simulink model "generic_mass_SoC_mu"  (R2025a)
settings: Solver=ode45  StartTime=0.0  StopTime=12  RelTol=1e-3  EnableMultiTasking=on
values from neighbouring files (symbols this model uses):
  Battery =     [Battery_A123_Pack_204s2p_Final.mat]
  cs_tyre = 2.0e5    (= 200000)    [mu_estimator_parameters.m]
  dOCV_dSoC = gradient(OCV, SoC_bp)    [SoCOcv.m]
  dR0 = gradient(R0, SoC_L)    [SoCOcv.m]
  eps_vx = 0.5    [mu_estimator_parameters.m]
  fz_max = 6000    [mu_estimator_parameters.m]
  fz_min = 300    [mu_estimator_parameters.m]
  h_cg = 0.55    [mu_estimator_parameters.m]
  lf = 1.214    [mu_estimator_parameters.m]
  lr = 1.505    [mu_estimator_parameters.m]
  r0 = 0.344    [mu_estimator_parameters.m]
  re_max = 0.33    [mu_estimator_parameters.m]
  re_min = 0.28    [mu_estimator_parameters.m]
  SoC_bp = Table_SoCvsOCV.LUT.SoC_percent    [SoCOcv.m]
  SoC_L = Battery.SOC_LUT    [SoCOcv.m]
  Table_SoCvsOCV = load("SoC_to_Voltage_LUT_10000-GON.mat")    [SoCOcv.m]
  tw_f = 1.571    [mu_estimator_parameters.m]
  tw_r = 1.581    [mu_estimator_parameters.m]
undefined symbols (not defined in the file or in its folder): DiscIntNeverNeededParam, Init_SoC
libraries: CarMaker4SL x41, simulink x1
(part 1 of 4)
settings Model: ModifiedByFormat=IPG  ExtModeAutoUpdateStatusClock=off  VariantFading=off  Creator=IPG  LastModifiedBy=IPG
settings SolverCC: AlgebraicLoopSolver=TrustRegion
settings DataIOCC: LimitDataPoints=on  SaveFormat=Array  SignalLoggingSaveFormat=ModelDataLogs  ReturnWorkspaceOutputs=off  SignalLoggingName=sigsOut
settings OptimizationCC: BooleanDataType=off  ReuseModelBlockBuffer=off  ExpressionDepthLimit=2147483647.0  InitFltsAndDblsToZero=on  LifeSpan=inf
settings DebuggingCC: SaveWithParameterizedLinksMsg=none  UnderspecifiedInitializationDetection=Classic  MergeDetectMultiDrivingBlocksExec=none  SignalResolutionControl=TryResolveAllWithWarning  MultiTaskDSMMsg=warning  MultiTaskCondExecSysMsg=none  FcnCallInpInsideContextMsg=warning  UnconnectedInputMsg=warning  UnconnectedOutputMsg=warning  UnconnectedLineMsg=warning  StateNameClashWarn=warning  SFUnexpectedBacktrackingDiag=warning  SFNoUnconditionalDefaultTransitionDiag=warning  ArithmeticOperatorsInVariantConditions=warning
settings HardwareCC: ProdBitPerPointer=32.0  ProdBitPerSizeT=32.0  ProdBitPerPtrDiffT=32.0  ProdLargestAtomicFloat=None  ProdIntDivRoundTo=Undefined  ProdEndianess=Unspecified  ProdWordSize=32.0  ProdHWDeviceType=32-bit Generic  TargetUnknown=on
settings ModelReferenceCC: EnableRefExpFcnMdlSchedulingChecks=on  PropagateSignalLabelsOutOfModel=off
settings SFSimCC: SimUseLocalCustomCode=off  CustomCodeUndefinedFunction=UseInterfaceOnly
settings RTWCC: RTWUseLocalCustomCode=off  GPUComputeCapability=3.5  DLArmComputeVersion=19.05
settings CodeAppCC: MaxIdLength=63.0  StateflowObjectComments=on
settings GRTTargetCC: TargetFcnLib=ansi_tfl_tmw.mat  TargetLangStandard=C89/C90 (ANSI)  CombineOutputUpdateFcns=off  GRTInterface=on
settings ConfigComp: CovMetricSettings=dw  CovSaveCumulativeToWorkspaceVar=on  CovSaveSingleToWorkspaceVar=on  CovExternalEMLEnable=off

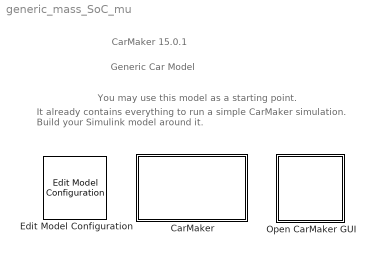
== system generic_mass_SoC_mu ==
  note: Generic Car Model
  note: You may use this model as a starting point.
  note: It already contains everything to run a simple CarMaker simulation.
      | Build your Simulink model around it.
  note: CarMaker 15.0.1
  CarMaker : Subsystem  TreatAsAtomicUnit=on
      mask Display: image(imread('CarMakerSys.png'));
  Edit Model Configuration : CarMaker4SL/Edit Model Configuration  SFunctionModules=''
  Open CarMaker GUI : Subsystem  LoadFcn=if ~length(which('cmself')), cmenv; end
      settings: OpenFcn=cmblockmagic('gui_fix_display'); CM_Simulink
      mask Display: image(imread('CarMakerGUI.png'));

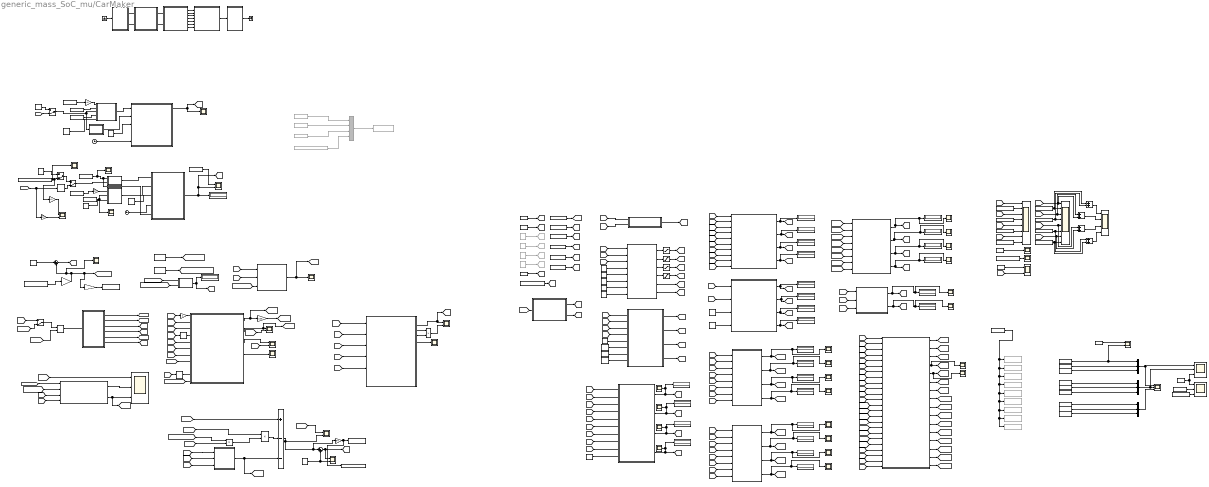
== system generic_mass_SoC_mu/CarMaker ==
  note: Data for Heavy Braking Tests
  note: Heavy Braking Test - Fx Comparison
  note: front_wheel_speed_from_motor
  note: SOC Estimator
  note: Mass and Slop Estimator
  note: Slope Estimator
  note: Mass estimation
  note: Current Input
  note: EXTENDED KALMAN FILTER SOC
  note: Internal resistance estimation
  note: Vt
  note: I.R
  note: Voltage of RC network
  note: ECM MODEL
  note: Terminal
      |  voltage
  note: OCV
  note: INIT
  note: SoC comparison
  note: Cell Capacity Calculation
  note: ECM LOOKUP TABLES
  note: cornering_detector
  note: Mu estimator - Motor Front - 2 Wheels Rear
  note: Outputs
  note: effective_radius_estimator
  note: vertical_load_estimator
  note: Inputs
  note: longitudinal_force_estimator
  note: slip_estimator
  note: mu_combined_estimator
  note: longitudinal_accel_correction
  note: lateral_force_estimator
  note: mu_long_estimator
  note: mu_lat_estimator
  Add : Sum  Inputs=+--
  Add{1..4} (4 alike) : Sum
  Battery total capacity (mAh)2 : Constant  Value=6000
  CM_FIRST : Subsystem
  CM_LAST : Subsystem
  COLOUMB COUNTING : Subsystem
  Clock1 : Clock
  Clock2 : Clock
  Constant : Constant  Value=0.343
  Constant1 : Constant  Value=1770.02
  Constant2 : Constant
  Constant3 : Constant  Value=0.75
  Constant32 : Constant  Value=lf
  Constant33 : Constant  Value=lr
  Constant34 : Constant  Value=h_cg
  Constant35 : Constant  Value=r0
  Constant36 : Constant  Value=cs_tyre
  Constant37 : Constant  Value=re_min
  Constant38 : Constant  Value=re_max
  Constant39 : Constant  Value=eps_vx
  Constant4 : Constant  Value=0
  Constant46 : Constant  Commented=on  Value=1770
  Constant47 : Constant  Commented=on
  Constant48 : Constant  Commented=on  Value=0
  Constant49 : Constant  Value=tw_r
  Constant5 : Constant  Value=1900
  Constant50 : Constant  Value=tw_f
  Constant51 : Constant  Commented=on  Value=0.15
  Constant6 : Constant  Value=0.343
  Constant7 : Constant  Value=lf
  Constant8 : Constant  Value=lr
  Delay : Delay  DelayLength=1  InputProcessing=Columns as channels (frame based)
  Delay1 : Delay  DelayLength=1  InitialConditionSource=Input port  InitialCondition=Init_SoC  InputProcessing=Columns as channels (frame based)
      settings: InputPortMap=u0,p4
  Delay2 : Delay  DelayLength=1  InputProcessing=Columns as channels (frame based)
  Delay3 : Delay  DelayLength=1  InputProcessing=Columns as channels (frame based)
  Display{,1..13,24..37} (28 alike) : Display
  DrivMan : Subsystem
  EKF : MATLAB Function  TreatAsAtomicUnit=on
  Factor internal Resistance : Constant  Value=1.5
  From Workspace : FromWorkspace  VariableName=dryunload
  From Workspace1 : FromWorkspace  VariableName=dryload
  From Workspace2 : FromWorkspace  VariableName=wetunload
  From Workspace3 : FromWorkspace  VariableName=wetload
  From Workspace4 : FromWorkspace  VariableName=dryload1
  From Workspace5 : FromWorkspace  VariableName=wetload1
  From Workspace6 : FromWorkspace  VariableName=iceunload
  From Workspace7 : FromWorkspace  VariableName=iceload
  From Workspace8 : FromWorkspace  VariableName=iceload1
  Gain : Gain  Gain=180/pi
  Gain1 : Gain  Gain=10.65
  Gain2 : Gain  Gain=10.65
  Gain3 : Gain  Gain=180/pi
  Gain4 : Gain  Gain=3/180.9
  Gain5 : Gain  Gain=100
  Gain6 : Gain
  Gain7 : Gain  Gain=94
  Gain8 : Gain  Gain=180.9/3
  Goto112 : Goto  Commented=on  GotoTag=mhat  TagVisibility=global
  Goto123 : Goto  Commented=on  GotoTag=brake  TagVisibility=global
  Goto127 : Goto  Commented=on  GotoTag=throttle  TagVisibility=global
  Goto97 : Goto  Commented=on  GotoTag=beta  TagVisibility=global
  Ground : Ground
  INTERNAL RESISTANCE ESTIMATION : MATLAB Function  TreatAsAtomicUnit=on
  IPG Vehicle : Subsystem
  MATLAB Function : MATLAB Function  TreatAsAtomicUnit=on
  MATLAB Function1 : MATLAB Function  TreatAsAtomicUnit=on
  MATLAB Function17 : MATLAB Function  TreatAsAtomicUnit=on
  MATLAB Function2 : MATLAB Function  TreatAsAtomicUnit=on
  MATLAB Function23 : MATLAB Function  TreatAsAtomicUnit=on
  MATLAB Function24 : MATLAB Function  TreatAsAtomicUnit=on
  MATLAB Function26 : MATLAB Function  TreatAsAtomicUnit=on
  MATLAB Function27 : MATLAB Function  TreatAsAtomicUnit=on
  MATLAB Function28 : MATLAB Function  TreatAsAtomicUnit=on
  MATLAB Function29 : MATLAB Function  TreatAsAtomicUnit=on
  MATLAB Function3 : MATLAB Function  TreatAsAtomicUnit=on
  MATLAB Function30 : MATLAB Function  TreatAsAtomicUnit=on
  MATLAB Function4 : MATLAB Function  TreatAsAtomicUnit=on
  MATLAB Function5 : MATLAB Function  TreatAsAtomicUnit=on
  MATLAB Function6 : MATLAB Function  TreatAsAtomicUnit=on
  MATLAB Function7 : MATLAB Function  TreatAsAtomicUnit=on
  MATLAB Function8 : MATLAB Function  TreatAsAtomicUnit=on
  MATLAB Function9 : MATLAB Function  TreatAsAtomicUnit=on
  Manual Switch{,1..3} (4 alike) : ManualSwitch  CurrentSetting=0
  Mass Estimator : MATLAB Function  TreatAsAtomicUnit=on
  Measurement Error : RandomNumber  Variance=0.00001  Seed=18618  SampleTime=0.01
  Mux : Mux  Inputs=3
  Mux1 : Mux  Inputs=3
  Mux2 : Mux  Inputs=3
  Mux3 : Mux  Commented=on
  Parameter updating : Subsystem
  Process Error : RandomNumber  Variance=0.1  Seed=234513235  SampleTime=0.01
  Product : Product
  Product1 : Product
  RC network subsystem : Subsystem
  Read CM Dict{,3,10,12,25,32} (6 alike) : CarMaker4SL/Read CM Dict  xname=Car.ax  xsync=off  xstime=Continuous
  Read CM Dict1 : CarMaker4SL/Read CM Dict  xname=Car.vx  xsync=off  xstime=Continuous
  Read CM Dict11 : CarMaker4SL/Read CM Dict  xname=Vhcl.FR.rotv  xsync=off  xstime=Continuous
  Read CM Dict13 : CarMaker4SL/Read CM Dict  xname=Vhcl.FL.rotv  xsync=off  xstime=Continuous
  Read CM Dict14 : CarMaker4SL/Read CM Dict  xname=Vhcl.FR.rotv  xsync=off  xstime=Continuous
  Read CM Dict15 : CarMaker4SL/Read CM Dict  xname=Vhcl.RL.rotv  xsync=off  xstime=Continuous
  Read CM Dict16 : CarMaker4SL/Read CM Dict  xname=Vhcl.RR.rotv  xsync=off  xstime=Continuous
  Read CM Dict17 : CarMaker4SL/Read CM Dict  xname=Vhcl.FL.Fz  xsync=off  xstime=Continuous
  Read CM Dict18 : CarMaker4SL/Read CM Dict  xname=PT.Motor.rotv  xsync=off  xstime=Continuous
  Read CM Dict19 : CarMaker4SL/Read CM Dict  xname=Vhcl.FR.Fz  xsync=off  xstime=Continuous
  Read CM Dict2 : CarMaker4SL/Read CM Dict  xname=PT.Motor.Trq  xsync=off  xstime=Continuous
  Read CM Dict20 : CarMaker4SL/Read CM Dict  xname=Vhcl.RL.rotv  xsync=off  xstime=Continuous
  Read CM Dict21 : CarMaker4SL/Read CM Dict  xname=Vhcl.RR.rotv  xsync=off  xstime=Continuous
  Read CM Dict22 : CarMaker4SL/Read CM Dict  xname=Vhcl.RL.Fz  xsync=off  xstime=Continuous
  Read CM Dict23 : CarMaker4SL/Read CM Dict  xname=Vhcl.RR.Fz  xsync=off  xstime=Continuous
  Read CM Dict24 : CarMaker4SL/Read CM Dict  xname=Car.ay  xsync=off  xstime=Continuous
  Read CM Dict26 : CarMaker4SL/Read CM Dict  xname=Car.Road.Route.LongSlope  xsync=off  xstime=Continuous
  Read CM Dict27 : CarMaker4SL/Read CM Dict  xname=Car.Road.Route.LongSlope  xsync=off  xstime=Continuous
  Read CM Dict28 : CarMaker4SL/Read CM Dict  xname=Car.ay  xsync=off  xstime=Continuous
  Read CM Dict29 : CarMaker4SL/Read CM Dict  xname=Vhcl.Steer.Ang  xsync=off  xstime=Continuous
  Read CM Dict30 : CarMaker4SL/Read CM Dict  xname=Car.YawRate  xsync=off  xstime=Continuous
  Read CM Dict31 : CarMaker4SL/Read CM Dict  xname=Car.SideSlipAngle  xsync=off  xstime=Continuous
  Read CM Dict33 : CarMaker4SL/Read CM Dict  xname=Car.vx  xsync=off  xstime=Continuous
  Read CM Dict34 : CarMaker4SL/Read CM Dict  Commented=on  xname=PT.Motor.Trq  xsync=off  xstime=Continuous
  Read CM Dict35 : CarMaker4SL/Read CM Dict  Commented=on  xname=Car.vx  xsync=off  xstime=Continuous
  Read CM Dict36 : CarMaker4SL/Read CM Dict  Commented=on  xname=Car.ax  xsync=off  xstime=Continuous
  Read CM Dict37 : CarMaker4SL/Read CM Dict  Commented=on  xname=Car.Road.Route.LongSlope  xsync=off  xstime=Continuous
  Read CM Dict4 : CarMaker4SL/Read CM Dict  xname=Car.Road.Route.LongSlope  xsync=off  xstime=Continuous
  Read CM Dict5 : CarMaker4SL/Read CM Dict  xname=PT.Motor.Trq  xsync=off  xstime=Continuous
  Read CM Dict6 : CarMaker4SL/Read CM Dict  xname=Car.vx  xsync=off  xstime=Continuous
  Read CM Dict7 : CarMaker4SL/Read CM Dict  xname=Vhcl.FR.Fx  xsync=off  xstime=Continuous
  Read CM Dict8 : CarMaker4SL/Read CM Dict  xname=PT.Motor.Trq  xsync=off  xstime=Continuous
  Read CM Dict9 : CarMaker4SL/Read CM Dict  xname=PT.BattHV.Current  xsync=off  xstime=Continuous
  Saturation{4..7} (4 alike) : Saturate  UpperLimit=fz_max  LowerLimit=fz_min
  Scope{,1..2,4,6,9,13,15..25,29..38,42,44} (30 alike) : Scope
      Scope settings: ActiveDisplayYMinimum=-1  ActiveDisplayYMaximum=1
      Scope1 settings: ActiveDisplayYMinimum=-1  ActiveDisplayYMaximum=1
      Scope13 settings: ActiveDisplayYMinimum=-0.0040490561765422206  ActiveDisplayYMaximum=0.0023870747364762024  DataLoggingVariableName=ScopeData13
      Scope15 settings: ActiveDisplayYMinimum=5.267786429043011  ActiveDisplayYMaximum=6.0813570634396656  DataLoggingVariableName=ScopeData15
      Scope16 settings: ActiveDisplayYMinimum=-0.78309060543519626  ActiveDisplayYMaximum=0.78396172750172144  DataLoggingVariableName=ScopeData18
      Scope17 settings: ActiveDisplayYMinimum=-1  ActiveDisplayYMaximum=1  DataLoggingVariableName=ScopeData19
      Scope18 settings: ActiveDisplayYMinimum=-1  ActiveDisplayYMaximum=1  DataLoggingVariableName=ScopeData20
      Scope19 settings: ActiveDisplayYMinimum=-1  ActiveDisplayYMaximum=1  DataLoggingVariableName=ScopeData21
      Scope2 settings: ActiveDisplayYMinimum=-1  ActiveDisplayYMaximum=1  DataLoggingVariableName=ScopeData2
      Scope20 settings: ActiveDisplayYMinimum=-0.78309060543519626  ActiveDisplayYMaximum=0.78396172750172144  DataLoggingVariableName=ScopeData22
      Scope21 settings: ActiveDisplayYMinimum=-1  ActiveDisplayYMaximum=1  DataLoggingVariableName=ScopeData23
      Scope22 settings: ActiveDisplayYMinimum=-1  ActiveDisplayYMaximum=1  DataLoggingVariableName=ScopeData24
      Scope23 settings: ActiveDisplayYMinimum=-1  ActiveDisplayYMaximum=1  DataLoggingVariableName=ScopeData25
      Scope24 settings: ActiveDisplayYMinimum=-7189.1945849733847  ActiveDisplayYMaximum=6347.4205470208444  DataLoggingVariableName=ScopeData26
      Scope25 settings: ActiveDisplayYMinimum=-3261.1629631477726  ActiveDisplayYMaximum=457.08980839058904  DataLoggingVariableName=ScopeData27
      Scope29 settings: ActiveDisplayYMinimum=-0.092654151933100309  ActiveDisplayYMaximum=0.77993922328861376  DataLoggingVariableName=ScopeData31
      Scope30 settings: ActiveDisplayYMinimum=-1  ActiveDisplayYMaximum=1  DataLoggingVariableName=ScopeData32
      Scope31 settings: ActiveDisplayYMinimum=-1  ActiveDisplayYMaximum=1  DataLoggingVariableName=ScopeData33
      Scope32 settings: ActiveDisplayYMinimum=-1  ActiveDisplayYMaximum=1  DataLoggingVariableName=ScopeData34
      Scope33 settings: DataLoggingVariableName=ScopeData35
      Scope34 settings: DataLoggingVariableName=ScopeData36
      Scope35 settings: DataLoggingVariableName=ScopeData37
      Scope36 settings: DataLoggingVariableName=ScopeData38
      Scope37 settings: ActiveDisplayYMinimum=-1  ActiveDisplayYMaximum=1  DataLoggingVariableName=ScopeData39
      Scope38 settings: ActiveDisplayYMinimum=-0.0655570660830278  ActiveDisplayYMaximum=0.59001359474725035  DataLoggingVariableName=ScopeData40
      Scope4 settings: ActiveDisplayYMinimum=0.17650245012519925  ActiveDisplayYMaximum=0.22445297416691398  DataLoggingVariableName=ScopeData6
      Scope42 settings: ActiveDisplayYMinimum=-1  ActiveDisplayYMaximum=1  DataLoggingVariableName=ScopeData44
      Scope44 settings: ActiveDisplayYMinimum=-1  ActiveDisplayYMaximum=1  DataLoggingVariableName=ScopeData46
      Scope6 settings: ActiveDisplayYMinimum=-7.6253012416574766  ActiveDisplayYMaximum=8.8462173056425879  DataLoggingVariableName=ScopeData4
      Scope9 settings: ActiveDisplayYMinimum=-0.0013929215683664009  ActiveDisplayYMaximum=0.0015298641956065784  DataLoggingVariableName=ScopeData8
  Scope{3,5,7..8,10..12,39,43} (9 alike) : Scope  NumInputPorts=2
      Scope10 settings: ActiveDisplayYMinimum=65.290304256240674  ActiveDisplayYMaximum=81.634785578223827  DataLoggingVariableName=ScopeData12
      Scope11 settings: ActiveDisplayYMinimum=0.0023982019976572207  ActiveDisplayYMaximum=0.002548408512625157  DataLoggingVariableName=ScopeData11
      Scope12 settings: ActiveDisplayYMinimum=-0.56498027572656229  ActiveDisplayYMaximum=4.9570490949911772  DataLoggingVariableName=ScopeData10
      Scope3 settings: ActiveDisplayYMinimum=1671.5980824561561  ActiveDisplayYMaximum=1724.2201262046208  DataLoggingVariableName=ScopeData5
      Scope39 settings: ActiveDisplayYMinimum=-1  ActiveDisplayYMaximum=1  DataLoggingVariableName=ScopeData41
      Scope43 settings: ActiveDisplayYMinimum=-21.798623721322567  ActiveDisplayYMaximum=18.483609956058363  DataLoggingVariableName=ScopeData45
      Scope5 settings: ActiveDisplayYMinimum=1.9265881549094703  ActiveDisplayYMaximum=4.0763345822165622  DataLoggingVariableName=ScopeData3
      Scope7 settings: ActiveDisplayYMinimum=3.7961685683353883  ActiveDisplayYMaximum=4.0277331935579088  DataLoggingVariableName=ScopeData7
      Scope8 settings: ActiveDisplayYMinimum=-0.11005098491461757  ActiveDisplayYMaximum=0.33783186441057322  DataLoggingVariableName=ScopeData9
  Scope{14,26..28} (4 alike) : Scope  NumInputPorts=3
      Scope14 settings: ActiveDisplayYMinimum=77.508392623156581  ActiveDisplayYMaximum=80.277220204122059  DataLoggingVariableName=ScopeData14
      Scope26 settings: ActiveDisplayYMinimum=-6904.8747954168166  ActiveDisplayYMaximum=5352.9283821189529  DataLoggingVariableName=ScopeData28
      Scope27 settings: ActiveDisplayYMinimum=-14.214999613778026  ActiveDisplayYMaximum=6.4649955098955347  DataLoggingVariableName=ScopeData29
      Scope28 settings: ActiveDisplayYMinimum=-10103.459891915962  ActiveDisplayYMaximum=5366.5694146923006  DataLoggingVariableName=ScopeData30
  Scope40 : Scope  NumInputPorts=8
      settings: ActiveDisplayYMinimum=-7.925692503758305  ActiveDisplayYMaximum=71.331065439918262  DataLoggingVariableName=ScopeData42
  Scope41 : Scope  NumInputPorts=8
      settings: ActiveDisplayYMinimum=1521.5777290365256  ActiveDisplayYMaximum=7221.6093076040352  DataLoggingVariableName=ScopeData43
  Scope45 : Scope  NumInputPorts=4
      settings: ActiveDisplayYMinimum=4074.5734716038833  ActiveDisplayYMaximum=14328.60737357984  DataLoggingVariableName=ScopeData47
  Slope estimator : MATLAB Function  TreatAsAtomicUnit=on
  Sum : Sum  Inputs=|++
  Sum2 : Sum  Inputs=|++
  Terminator : Terminator
  To Workspace : ToWorkspace  VariableName=I_cm_real  SaveFormat=Timeseries  SampleTime=-1
  To Workspace1 : ToWorkspace  VariableName=V_cm_real  SaveFormat=Timeseries  SampleTime=-1
  To Workspace10 : ToWorkspace  Commented=on  VariableName=iceload1  SaveFormat=Timeseries  SampleTime=-1
  To Workspace11 : ToWorkspace  Commented=on  VariableName=MK_DataCM  SaveFormat=Timeseries  SampleTime=-1
  To Workspace2 : ToWorkspace  Commented=on  VariableName=dryload  SaveFormat=Timeseries  SampleTime=-1
  To Workspace3 : ToWorkspace  Commented=on  VariableName=dryunload  SaveFormat=Timeseries  SampleTime=-1
  To Workspace4 : ToWorkspace  Commented=on  VariableName=wetunload  SaveFormat=Timeseries  SampleTime=-1
  To Workspace5 : ToWorkspace  Commented=on  VariableName=wetload  SaveFormat=Timeseries  SampleTime=-1
  To Workspace6 : ToWorkspace  Commented=on  VariableName=dryload1  SaveFormat=Timeseries  SampleTime=-1
  To Workspace7 : ToWorkspace  Commented=on  VariableName=wetload1  SaveFormat=Timeseries  SampleTime=-1
  To Workspace8 : ToWorkspace  Commented=on  VariableName=iceload  SaveFormat=Timeseries  SampleTime=-1
  To Workspace9 : ToWorkspace  Commented=on  VariableName=iceunload  SaveFormat=Timeseries  SampleTime=-1
  VehicleControl : Subsystem
  Write CM Dict1 : CarMaker4SL/Write CM Dict  xname=PT.BattHV.Volt_oc  xsync=off
  multiply : Product  Inputs=**
  tag scope: HL=global, R0=global, Uoc=global, ax=global, ax_eff=global, ay=global, corner=global, dUoc_dSoc=global, fx_fl=global, fx_fr=global, fx_front=global, fx_rear=global, fx_rl=global, fx_rr=global, fy_fl=global, fy_fr=global, fy_front=global, fy_rear=global, fy_rl=global, fy_rr=global, fz_fl=global, fz_fr=global, fz_front=global, fz_rear=global, fz_rl=global, fz_rr=global, mu=global, mu_fl=global, mu_fr=global, mu_front=global, mu_lat=global, mu_lat_fl=global, mu_lat_fr=global, mu_lat_front=global, mu_lat_rear=global, mu_lat_rl=global, mu_lat_rr=global, mu_long=global, mu_long_fl=global, mu_long_fr=global, mu_long_front=global, mu_long_rear=global, mu_long_rl=global, mu_long_rr=global, mu_rear=global, mu_rl=global, mu_rr=global, om_fl=global, om_fr=global, om_front=global, om_rl=global, om_rr=global, re_fl=global, re_fr=global, re_rl=global, re_rr=global, slip=global, slipAng=global, slip_fl=global, slip_fr=global, slip_front=global, slip_rear=global, slip_rl=global, slip_rr=global, slope=global, steer=global, vx=global, yaw_r=global
  wires:
  DrivMan/2(DrivMan.Out) -> VehicleControl/2(DrivMan.In)
  DrivMan/1(Sync_Out) -> VehicleControl/1(Sync_In)
  CM_FIRST/2(Env.Misc) -> DrivMan/2(Env.Misc)
  CM_FIRST/1(Sync_Out) -> DrivMan/1(Sync_In)
  CM_LAST/1(Sync_Out) -> Terminator/1
  Ground/1 -> CM_FIRST/1(Sync_In)
  IPG Vehicle/1(Sync_Out) -> CM_LAST/1(Sync_In)
  VehicleControl/1(Sync_Out) -> IPG Vehicle/1(Sync_In)
  VehicleControl/3(VhclCtrl.Steering) -> IPG Vehicle/3(VhclCtrl.Steering)
  VehicleControl/4(Vhcl.Wheel.In) -> IPG Vehicle/4(Vhcl.Wheel.In)
  VehicleControl/5(Vhcl.Misc) -> IPG Vehicle/5(Vhcl.Misc)
  VehicleControl/6(VhclCtrl.Brake) -> IPG Vehicle/6(VhclCtrl.Brake)
  VehicleControl/7(VhclCtrl.PT) -> IPG Vehicle/7(VhclCtrl.PT)
  VehicleControl/2(Vhcl.Model.Source) -> IPG Vehicle/2(Vhcl.Model.Source)
  [mhat] -> Manual Switch2/2
  Read CM Dict2/1 -> Gain2/1
  Slope estimator/1(theta2_hat) -> Scope4/1, [beta]
  Constant3/1 -> Slope estimator/3(lambda2)
  Constant5/1 -> Manual Switch2/1
  Manual Switch2/1 -> MATLAB Function5/3(mhat), MATLAB Function6/1(mhat)
  Read CM Dict1/1 -> MATLAB Function5/2(vx)
  MATLAB Function5/1(y2) -> Slope estimator/1(y2)
  Clock1/1 -> Slope estimator/5(t)
  MATLAB Function6/1(phi2) -> Slope estimator/2(phi2)
  Read CM Dict/1 -> MATLAB Function5/4(ax)
  Clock2/1 -> Mass Estimator/4(t)
  Manual Switch/1 -> MATLAB Function2/2(beta)
  Read CM Dict4/1 -> Scope1/1, Gain3/1, Manual Switch1/2
  Mass Estimator/1(m_hat) -> [mhat], Scope3/2, Display/1
  Constant4/1 -> Manual Switch1/1
  MATLAB Function3/1(phi) -> Mass Estimator/2(phi)
  Read CM Dict5/1 -> Gain1/1
  Delay/1 -> Manual Switch/2
  Constant2/1 -> Mass Estimator/3(lambda)
  Manual Switch1/1 -> Manual Switch/1
  Read CM Dict6/1 -> Scope/1, MATLAB Function3/2(vx)
  MATLAB Function2/1(y) -> Mass Estimator/1(y)
  [beta] -> Gain/1, Delay/1
  Read CM Dict3/1 -> Scope2/1, Mass Estimator/5(ax), MATLAB Function2/1(ax)
  Gain1/1 -> MATLAB Function3/1(T_tq)
  Gain2/1 -> MATLAB Function5/1(Tq)
  Constant1/1 -> Scope3/1
  Constant6/1 -> MATLAB Function3/3(re)
  Gain/1 -> Scope5/2
  Gain3/1 -> Scope5/1
  Sum2/1 -> [Current]
  Read CM Dict9/1 -> Gain4/1
  Gain4/1 -> Scope6/1, Sum2/2, Gain8/1, [current_real]
  Process Error/1 -> Sum2/1
  [Vp_real] -> Scope8/2  "Vp_real"
  [Uoc] -> EKF/3(Uoc)
  EKF/3(ul_hat) -> Scope7/1  "vt_hat"
  Delay2/1 -> EKF/10(Qcap_est)
  [Vt] -> EKF/2(UL_meas)
  [R0] -> EKF/5(R0nom)
  EKF/2(u1_hat) -> [u1_hat], Scope8/1  "Vp_hat"
  INTERNAL RESISTANCE ESTIMATION/2(innov_theta) -> Scope13/1
  [MaxBatteryCap] -> EKF/11(Qnom)
  [Uoc] -> INTERNAL RESISTANCE ESTIMATION/3(Uoc)
  [C1] -> EKF/7(C1)
  [R0] -> Product1/1
  [Vt] -> Scope7/2  "vt_real"
  Delay3/1 -> EKF/4(R0_est)
  EKF/4(innov) -> Scope9/1
  Gain6/1 -> EKF/1(I)
  [Current] -> Gain6/1
  [u1_hat] -> INTERNAL RESISTANCE ESTIMATION/5(u1_hat)
  [R0] -> INTERNAL RESISTANCE ESTIMATION/4(R0_init)
  [Vt] -> INTERNAL RESISTANCE ESTIMATION/2(UL_meas)
  Product1/1 -> Scope11/2  "real_R0"
  INTERNAL RESISTANCE ESTIMATION/1(R0_hat) -> [R0_hat], Scope11/1  "R0 hat"
  [dUoc_dSoc] -> EKF/8(dUoc_dSoc)
  [Facto_Internal_Resistance] -> Product1/2
  [R0_hat] -> Delay3/1
  [R1] -> EKF/6(R1)
  Gain5/1 -> [SoC]
  [Q_est] -> Delay2/1
  EKF/1(soc_hat) -> [SoC_hat], Gain5/1
  [Current] -> INTERNAL RESISTANCE ESTIMATION/1(I)
  [C1] -> RC network subsystem/3(" C1")
  Product/1 -> multiply/2
  [R1] -> RC network subsystem/2(R1)
  [current_real] -> multiply/1
  [Facto_Internal_Resistance] -> Product/1
  [Uoc] -> Add/1
  Add/1 -> Gain7/1, Sum/1, Scope10/2
  [R0] -> Product/2
  [current_real] -> RC network subsystem/1(current (A))
  Measurement Error/1 -> Sum/2, Scope12/2
  RC network subsystem/1(V1) -> [Vp_real], Add/3
  multiply/1 -> Add/2
  [SoC] -> Scope10/1
  MATLAB Function4/1(Q_real) -> [Q_real], Display1/1
  [Facto_Internal_Resistance] -> MATLAB Function4/2(factor_internal_resistance)
  Factor internal Resistance/1 -> [Facto_Internal_Resistance]
  [MaxBatteryCap] -> MATLAB Function4/1(Qmax)
  Battery total capacity (mAh)2/1 -> [MaxBatteryCap]
  [Q_real] -> COLOUMB COUNTING/4(Q_real)
  COLOUMB COUNTING/2(Col COUNT) -> Scope14/3, [SoC_Col]  "Coloumb Counting"
  [MaxBatteryCap] -> COLOUMB COUNTING/2(Qmax)
  [current_real] -> COLOUMB COUNTING/1(current real)
  [SoC] -> Scope14/1  "EKF"
  [Current] -> COLOUMB COUNTING/3(current real1)
  COLOUMB COUNTING/1(Real Soc) -> Scope14/2  "Real SoC"
  MATLAB Function/1(C_batt) -> [Q_est], Scope15/1
  [MaxBatteryCap] -> MATLAB Function/3(C_init)
  [R0] -> MATLAB Function/2(R_init)
  [R0_hat] -> MATLAB Function/1(R_batt)
  Gain8/1 -> To Workspace/1
  Sum/1 -> Scope12/1, [Vt]
  Parameter updating/2(Ro) -> [R0]
  Manual Switch3/1 -> Delay1/1
  Parameter updating/1(Voc) -> [Uoc]
  Parameter updating/4(C1) -> [C1]
  [SoC_Col] -> Manual Switch3/2
  Delay1/1 -> Parameter updating/1(SoC)
  [SoC] -> Manual Switch3/1
  Parameter updating/6(dR0) -> [dR0]
  Parameter updating/5(dVoc) -> [dUoc_dSoc]
  [Init_SoC] -> Delay1/2
  Parameter updating/3(R1) -> [R1]
  Gain7/1 -> Write CM Dict1/1, To Workspace1/1
  Constant/1 -> MATLAB Function5/5(re)
  Read CM Dict29/1 -> [steer]
  Read CM Dict31/1 -> [slipAng]
  Read CM Dict30/1 -> [yaw_r]
  Read CM Dict28/1 -> [ay]
  MATLAB Function27/2(high_lateral_flag) -> [HL], Display29/1, Scope38/1
  MATLAB Function27/1(cornering_flag) -> [corner], Display28/1, Scope37/1
  [ay] -> MATLAB Function27/1(steer)
  [slipAng] -> MATLAB Function27/2(ay)
  [steer] -> MATLAB Function27/3(slip_angle)
  Read CM Dict18/1 -> [om_front]
  Read CM Dict20/1 -> [om_rl]
  Read CM Dict21/1 -> [om_rr]
  Read CM Dict33/1 -> [vx]
  Read CM Dict32/1 -> [ax]
  [fz_rl] -> MATLAB Function29/3(fz_rl)
  [re_fr] -> MATLAB Function30/7(re_fr)
  [slip_rl] -> MATLAB Function26/3(slip_rl)
  MATLAB Function26/2(slip_rear_avg) -> [slip_rear]
  Constant46/1 -> Goto112/1
  Constant51/1 -> Goto97/1
  Constant48/1 -> Goto127/1
  Constant39/1 -> MATLAB Function30/10(eps_vx)
  Constant47/1 -> Goto123/1
  Saturation4/1 -> [fz_fl]
  MATLAB Function26/8(mu_long_front_avg) -> [mu_long_front]
  [re_rl] -> MATLAB Function30/8(re_rl)
  Constant38/1 -> MATLAB Function29/8(re_max)
  [ax] -> MATLAB Function17/1(ax)
  MATLAB Function17/1(ax_eff) -> [ax_eff]
  [gas] -> MATLAB Function23/10(throttle_cmd)
  [slip_rr] -> MATLAB Function26/4(slip_rr)
  [re_rr] -> MATLAB Function30/9(re_rr)
  [mu_long_rr] -> MATLAB Function24/4(mu_long_rr)
  MATLAB Function23/4(fx_rr) -> Display25/1, [fx_rr]
  [slip_fl] -> MATLAB Function26/1(slip_fl)
  Saturation6/1 -> [fz_rl]
  MATLAB Function30/1(slip_fl) -> [slip_fl], Display34/1, Scope36/1
  MATLAB Function23/3(fx_rl) -> Display24/1, [fx_rl]
  MATLAB Function23/2(fx_fr) -> Display27/1, [fx_fr]
  MATLAB Function26/7(fy_rear_total) -> [fy_rear]
  [vx] -> MATLAB Function30/5(omega_rr)
  [slip_fr] -> MATLAB Function26/2(slip_fr)
  MATLAB Function24/4(mu_comb_rr) -> [mu_rr], Display33/1, Scope32/1
  Saturation7/1 -> [fz_rr]
  Saturation5/1 -> [fz_fr]
  [mu_long_rl] -> MATLAB Function24/3(mu_long_rl)
  [mu_long_fl] -> MATLAB Function24/1(mu_long_fl)
  Constant35/1 -> MATLAB Function29/5(r0)
  [fz_fl] -> MATLAB Function29/1(fz_fl)
  [fz_rr] -> MATLAB Function29/4(fz_rr)
  Constant37/1 -> MATLAB Function29/7(re_min)
  [fz_fr] -> MATLAB Function29/2(fz_fr)
  Constant36/1 -> MATLAB Function29/6(cs_tyre)
  MATLAB Function30/3(slip_rl) -> [slip_rl], Display35/1, Scope34/1
  [om_fl] -> MATLAB Function30/1(vx)
  [mu_lat_rl] -> MATLAB Function24/7(mu_lat_rl)
  MATLAB Function26/3(slip_vehicle_avg) -> [slip]
  MATLAB Function29/1(re_fl) -> [re_fl]
  MATLAB Function29/4(re_rr) -> [re_rr]
  MATLAB Function26/6(fy_front_total) -> [fy_front]
  MATLAB Function29/3(re_rl) -> [re_rl]
  [om_rr] -> MATLAB Function30/4(omega_rl)
  MATLAB Function29/2(re_fr) -> [re_fr]
  MATLAB Function23/1(fx_fl) -> Display26/1, [fx_fl]
  MATLAB Function24/1(mu_comb_fl) -> [mu_fl], Display30/1, Scope29/1
  [re_fl] -> MATLAB Function30/6(re_fl)
  MATLAB Function24/3(mu_comb_rl) -> [mu_rl], Display32/1, Scope31/1
  [brake] -> MATLAB Function23/9(brake_cmd)
  [om_fr] -> MATLAB Function30/2(omega_fl)
  [om_rl] -> MATLAB Function30/3(omega_fr)
  MATLAB Function24/2(mu_comb_fr) -> [mu_fr], Display31/1, Scope30/1
  MATLAB Function30/2(slip_fr) -> [slip_fr], Display37/1, Scope35/1
  MATLAB Function30/4(slip_rr) -> [slip_rr], Display36/1, Scope33/1
  MATLAB Function26/1(slip_front_avg) -> [slip_front]
  MATLAB Function26/5(fx_rear_total) -> Scope25/1, [fx_rear]
  [mu_long_fr] -> MATLAB Function24/2(mu_long_fr)
  [mu_lat_rr] -> MATLAB Function24/8(mu_lat_rr)
  MATLAB Function26/10(mu_long_vehicle_avg) -> [mu_long]
  MATLAB Function26/9(mu_long_rear_avg) -> [mu_long_rear]
  [mu_lat_fl] -> MATLAB Function24/5(mu_lat_fl)
  [mu_lat_fr] -> MATLAB Function24/6(mu_lat_fr)
  [om_front] -> MATLAB Function1/1(omega_motor_f)
  MATLAB Function1/1(omega_fl) -> [om_fl]
  MATLAB Function1/2(omega_fr) -> [om_fr]
  Constant7/1 -> MATLAB Function7/3(lf)
  MATLAB Function7/1(fy_fl) -> Display4/1, [fy_fl]
  MATLAB Function7/2(fy_fr) -> Display5/1, [fy_fr]
  MATLAB Function7/3(fy_rl) -> Display2/1, [fy_rl]
  [ax_eff] -> MATLAB Function7/2(ay)
  MATLAB Function7/4(fy_rr) -> [fy_rr], Display3/1
  Constant8/1 -> MATLAB Function7/4(lr)
  [mhat] -> MATLAB Function7/1(mhat)
  [fx_fr] -> MATLAB Function8/2(fx_fr)
  [fx_fl] -> MATLAB Function8/1(fx_fl)
  [fx_rr] -> MATLAB Function8/4(fx_rr)
  [fz_fr] -> MATLAB Function8/6(fz_fr)
  MATLAB Function8/2(mu_long_fr) -> Scope17/1, Display7/1, [mu_long_fr]
  MATLAB Function8/3(mu_long_rl) -> Scope18/1, Display8/1, [mu_long_rl]
  MATLAB Function8/1(mu_long_fl) -> Scope16/1, Display6/1, [mu_long_fl]
  [fx_rl] -> MATLAB Function8/3(fx_rl)
  [fz_fl] -> MATLAB Function8/5(fz_fl)
  [fz_rl] -> MATLAB Function8/7(fz_rl)
  MATLAB Function8/4(mu_long_rr) -> Scope19/1, Display9/1, [mu_long_rr]
  [fz_rr] -> MATLAB Function8/8(fz_rr)
  [fz_rr] -> MATLAB Function9/8(fz_rr)
  MATLAB Function9/4(mu_lat_rr) -> [mu_lat_rr], Display13/1, Scope23/1
  [fz_rl] -> MATLAB Function9/7(fz_rl)
  [fz_fl] -> MATLAB Function9/5(fz_fl)
  [fy_rl] -> MATLAB Function9/3(fy_rl)
  MATLAB Function9/1(mu_lat_fl) -> [mu_lat_fl], Display10/1, Scope20/1
  MATLAB Function9/3(mu_lat_rl) -> [mu_lat_rl], Display12/1, Scope22/1
  MATLAB Function9/2(mu_lat_fr) -> [mu_lat_fr], Display11/1, Scope21/1
  [fz_fr] -> MATLAB Function9/6(fz_fr)
  [fy_rr] -> MATLAB Function9/4(fy_rr)
  [fy_fl] -> MATLAB Function9/1(fy_fl)
  [fy_fr] -> MATLAB Function9/2(fy_fr)
  [fx_fl] -> MATLAB Function26/5(fx_fl)
  [fx_fr] -> MATLAB Function26/6(fx_fr)
  [fx_rl] -> MATLAB Function26/7(fx_rl)
  [fx_rr] -> MATLAB Function26/8(fx_rr)
  [fy_fl] -> MATLAB Function26/9(fy_fl)
  [fy_fr] -> MATLAB Function26/10(fy_fr)
  [fy_rl] -> MATLAB Function26/11(fy_rl)
  [fy_rr] -> MATLAB Function26/12(fy_rr)
  [mu_fl] -> MATLAB Function26/21(mu_comb_fl)
  [mu_fr] -> MATLAB Function26/22(mu_comb_fr)
  [mu_rl] -> MATLAB Function26/23(mu_comb_rl)
  [mu_rr] -> MATLAB Function26/24(mu_comb_rr)
  [mu_long_fl] -> MATLAB Function26/13(mu_long_fl)
  [mu_long_fr] -> MATLAB Function26/14(mu_long_fr)
  [mu_long_rl] -> MATLAB Function26/15(mu_long_rl)
  [mu_long_rr] -> MATLAB Function26/16(mu_long_rr)
  [mu_lat_rr] -> MATLAB Function26/20(mu_lat_rr)
  [mu_lat_rl] -> MATLAB Function26/19(mu_lat_rl)
  [mu_lat_fr] -> MATLAB Function26/18(mu_lat_fr)
  [mu_lat_fl] -> MATLAB Function26/17(mu_lat_fl)
  MATLAB Function26/11(mu_lat_front_avg) -> [mu_lat_front]
  MATLAB Function26/12(mu_lat_rear_avg) -> [mu_lat_rear]
  MATLAB Function26/13(mu_lat_vehicle_avg) -> [mu_lat]
  MATLAB Function26/16(mu_comb_vehicle_avg) -> [mu]
  MATLAB Function26/15(mu_comb_rear_avg) -> [mu_rear]
  MATLAB Function26/14(mu_comb_front_avg) -> [mu_front]
  From Workspace/1 -> Scope39/2, Mux/1  "dry_unload"
  From Workspace1/1 -> Mux/2  "dry_load_400kg"
  From Workspace2/1 -> Mux1/1  "wet_unload"
  From Workspace3/1 -> Mux1/2  "wet_load_400kg"
  MATLAB Function26/4(fx_front_total) -> Scope24/1, [fx_front]
  From Workspace4/1 -> Mux/3  "dry_load_600kg"
  From Workspace5/1 -> Mux1/3  "wet_load_600kg"
  From Workspace6/1 -> Mux2/1  "ice_unload"
  From Workspace7/1 -> Mux2/2  "ice_load_400kg"
  From Workspace8/1 -> Mux2/3  "ice_load_600kg"
  Mux/1 -> Scope28/1, Scope26/1
  Mux1/1 -> Scope26/2, Scope28/2
  Mux2/1 -> Scope28/3
  Read CM Dict7/1 -> To Workspace2/1, To Workspace4/1, To Workspace5/1, To Workspace6/1, To Workspace7/1, To Workspace10/1, To Workspace8/1, To Workspace9/1, To Workspace3/1
  Read CM Dict10/1 -> Scope26/3, Scope27/1  "ax"
  Read CM Dict8/1 -> Scope27/2
  Read CM Dict11/1 -> Scope27/3
  Read CM Dict12/1 -> Scope39/1  "ax"
  [fz_rl] -> MATLAB Function23/7(fz_rl)
  [fz_rr] -> MATLAB Function23/8(fz_rr)
  [fz_fr] -> MATLAB Function23/6(fz_fr)
  [fz_fl] -> MATLAB Function23/5(fz_fl)
  [slip_fl] -> MATLAB Function23/1(slip_fl)
  [slip_fr] -> MATLAB Function23/2(slip_fr)
  [slip_rr] -> MATLAB Function23/4(slip_rr)
  [slip_rl] -> MATLAB Function23/3(slip_rl)
  [om_fl] -> Scope40/1  "om_fl"
  Read CM Dict13/1 -> Scope40/2  "fl"
  [om_fr] -> Scope40/3  "om_fr"
  Read CM Dict14/1 -> Scope40/4  "fr"
  [om_rl] -> Scope40/5  "om_rl"
  Read CM Dict15/1 -> Scope40/6  "rl"
  [om_rr] -> Scope40/7  "om_rr"
  Read CM Dict16/1 -> Scope40/8  "rr"
  Read CM Dict23/1 -> Add4/2, Scope41/8  "rr"
  [fz_rr] -> Scope41/7, Add2/2  "fz_rr"
  Read CM Dict22/1 -> Add4/1, Scope41/6  "rl"
  [fz_rl] -> Add2/1, Scope41/5  "fz_rl"
  Read CM Dict19/1 -> Add3/2, Scope41/4  "fr"
  [fz_fr] -> Add1/1, Scope41/3  "fz_fr"
  Read CM Dict17/1 -> Add3/1, Scope41/2  "fl"
  [fz_fl] -> Add1/2, Scope41/1  "fz_fl"
  Read CM Dict24/1 -> Scope42/1
  Read CM Dict25/1 -> Scope43/1
  [ax_eff] -> Scope43/2  "ax_eff"
  Read CM Dict26/1 -> [slope]
  [slope] -> MATLAB Function17/2(slope)
  Read CM Dict27/1 -> Scope44/1
  Add3/1 -> Scope45/1  "front_CM"
  Add1/1 -> Scope45/2  "front_est"
  Add2/1 -> Scope45/3  "rear_est"
  Add4/1 -> Scope45/4  "rear_CM"
  [mhat] -> MATLAB Function28/1(mhat)
  [ax_eff] -> MATLAB Function28/2(ax_eff)
  [ay] -> MATLAB Function28/3(ay)
  Constant32/1 -> MATLAB Function28/4(lf)
  Constant33/1 -> MATLAB Function28/5(lr)
  Constant34/1 -> MATLAB Function28/6(h_cg)
  Constant50/1 -> MATLAB Function28/7(tw_f)
  Constant49/1 -> MATLAB Function28/8(tw_r)
  MATLAB Function28/1(fz_fl) -> Saturation4/1
  MATLAB Function28/2(fz_fr) -> Saturation5/1
  MATLAB Function28/3(fz_rl) -> Saturation6/1
  MATLAB Function28/4(fz_rr) -> Saturation7/1
  MATLAB Function28/5(fz_front_total) -> [fz_front]
  MATLAB Function28/6(fz_rear_total) -> [fz_rear]
  Read CM Dict34/1 -> Mux3/1
  Read CM Dict35/1 -> Mux3/2
  Read CM Dict36/1 -> Mux3/3
  Read CM Dict37/1 -> Mux3/4
  Mux3/1 -> To Workspace11/1

== system generic_mass_SoC_mu/Open CarMaker GUI ==
  S-Function : S-Function  FunctionName=cm_gui  SFunctionDeploymentMode=off  EnableBusSupport=off

== system generic_mass_SoC_mu/CarMaker/CM_FIRST ==
  Sync_In : Inport
  BusCreator1 : BusCreator  Inputs=8
  BusCreator2 : BusCreator  Inputs=6
  Demux1 : Demux  Outputs=14
      settings: DisplayOption=none
  Environment : S-Function  FunctionName=CM_Sfun  Parameters='Environment'  SFunctionDeploymentMode=off  EnableBusSupport=off
  IoIn : S-Function  FunctionName=CM_Sfun  Parameters='IoIn'  SFunctionDeploymentMode=off  EnableBusSupport=off
  Terminator : Terminator
  Sync_Out : Outport  VectorParamsAs1DForOutWhenUnconnected=off
  Env.Misc : Outport  Port=2  VectorParamsAs1DForOutWhenUnconnected=off
  wires:
  BusCreator2/1 -> Terminator/1  "IF Environment (in)"
  BusCreator1/1 -> Env.Misc/1
  Demux1/14 -> BusCreator2/6  "Env sRoad"
  Demux1/13 -> BusCreator2/5  "Env PoI_GCS Elev"
  Demux1/12 -> BusCreator2/4  "Env PoI_GCS Lat"
  Demux1/11 -> BusCreator2/3  "Env PoI_GCS Long"
  Demux1/10 -> BusCreator2/2  "Env Time"
  Demux1/9 -> BusCreator2/1  "Env yDay"
  Demux1/8 -> BusCreator1/8  "Env WindVel_tot z"
  Demux1/7 -> BusCreator1/7  "Env WindVel_tot y"
  Demux1/6 -> BusCreator1/6  "Env WindVel_tot x"
  Demux1/5 -> BusCreator1/5  "Env SolarRadiation"
  Demux1/4 -> BusCreator1/4  "Env AirHumidity"
  Demux1/3 -> BusCreator1/3  "Env AirPressure"
  Demux1/2 -> BusCreator1/2  "Env AirDensity"
  Demux1/1 -> BusCreator1/1  "Env Temperature"
  Environment/2 -> Demux1/1
  Environment/1 -> Sync_Out/1
  IoIn/1 -> Environment/1
  Sync_In/1 -> IoIn/1

== system generic_mass_SoC_mu/CarMaker/CM_LAST ==
  Sync_In : Inport
  CM_User : S-Function  FunctionName=CM_Sfun  Parameters='CM_User'  SFunctionDeploymentMode=off  EnableBusSupport=off
  IoOut : S-Function  FunctionName=CM_Sfun  Parameters='IoOut'  SFunctionDeploymentMode=off  EnableBusSupport=off
  Sync_Out : Outport  VectorParamsAs1DForOutWhenUnconnected=off
  wires:
  IoOut/1 -> Sync_Out/1
  CM_User/1 -> IoOut/1
  Sync_In/1 -> CM_User/1

== system generic_mass_SoC_mu/CarMaker/COLOUMB COUNTING ==
  note: A . sec
  note: total capacity (mAh)
  note: mAh
  note: mAh
  note: A . sec
  note: total capacity (mAh)
  current real : Inport
  Qmax : Inport  Port=2
  current real1 : Inport  Port=3
  Q_real : Inport  Port=4
  (As) to (mAh)1 : Gain  Gain=1000/3600
  (As) to (mAh)2 : Gain  Gain=1000/3600
  Discrete-Time Integrator : DiscreteIntegrator  ICPrevOutput=DiscIntNeverNeededParam  ICPrevScaledInput=DiscIntNeverNeededParam
  Integrator : Integrator
  MATLAB Function1 : MATLAB Function  TreatAsAtomicUnit=on
  MATLAB Function2 : MATLAB Function  TreatAsAtomicUnit=on
  Relational Operator1 : RelationalOperator  Operator=<=  OutDataTypeStr=boolean  InputSameDT=off
  Relational Operator2 : RelationalOperator  Operator=<=  OutDataTypeStr=boolean  InputSameDT=off
  Stop Simulation1 : Stop
  Stop Simulation2 : Stop
  initial SOC (%)1 : Constant  Value=80
  initial SOC (%)2 : Constant  Value=80
  zero1 : Constant  Value=0
  zero2 : Constant  Value=0
  Real Soc : Outport
  Col COUNT : Outport  Port=2
  wires:
  zero1/1 -> Relational Operator1/2
  Relational Operator1/1 -> Stop Simulation1/1
  initial SOC (%)1/1 -> MATLAB Function1/2(SOC_init)
  current real/1 -> Integrator/1
  Q_real/1 -> MATLAB Function1/1(Ct)
  (As) to (mAh)1/1 -> MATLAB Function1/3(I)
  MATLAB Function1/1(SoC) -> Real Soc/1, Relational Operator1/1
  Integrator/1 -> (As) to (mAh)1/1
  zero2/1 -> Relational Operator2/2
  initial SOC (%)2/1 -> MATLAB Function2/2(SOC_init)
  MATLAB Function2/1(SoC) -> Col COUNT/1, Relational Operator2/1
  (As) to (mAh)2/1 -> MATLAB Function2/3(I)
  Relational Operator2/1 -> Stop Simulation2/1
  Qmax/1 -> MATLAB Function2/1(Ct)
  Discrete-Time Integrator/1 -> (As) to (mAh)2/1
  current real1/1 -> Discrete-Time Integrator/1

== system generic_mass_SoC_mu/CarMaker/DrivMan ==
  note: There's rarely a reason to override DrivMan signals.
      | Use the VehicleControl interface for this purpose.
  Sync_In : Inport
  Env.Misc : Inport  Port=2
  BusCreator : BusCreator  Inputs=20
  Demux : Demux  Outputs=20
      settings: DisplayOption=none
  DrivMan : S-Function  FunctionName=CM_Sfun  Parameters='DrivMan'  SFunctionDeploymentMode=off  EnableBusSupport=off
  Sync_Out : Outport  VectorParamsAs1DForOutWhenUnconnected=off
  DrivMan.Out : Outport  Port=2  VectorParamsAs1DForOutWhenUnconnected=off
  wires:
  Demux/8 -> BusCreator/8  "DrivMan SelectorCtrl"
  Demux/7 -> BusCreator/7  "DrivMan UserSignal4"
  Demux/6 -> BusCreator/6  "DrivMan UserSignal3"
  Demux/5 -> BusCreator/5  "DrivMan UserSignal2"
  Demux/4 -> BusCreator/4  "DrivMan UserSignal1"
  Demux/3 -> BusCreator/3  "DrivMan UserSignal0"
  Demux/2 -> BusCreator/2  "DrivMan Key"
  Demux/1 -> BusCreator/1  "DrivMan SST"
  Env.Misc/1 -> DrivMan/2
  Sync_In/1 -> DrivMan/1
  DrivMan/1 -> Sync_Out/1
  BusCreator/1 -> DrivMan.Out/1
  DrivMan/2 -> Demux/1
  Demux/9 -> BusCreator/9  "DrivMan DigitalSelectorCtrl0"
  Demux/10 -> BusCreator/10  "DrivMan DigitalSelectorCtrl1"
  Demux/11 -> BusCreator/11  "DrivMan DigitalSelectorCtrl2"
  Demux/20 -> BusCreator/20  "DrivMan Steering Trq"
  Demux/19 -> BusCreator/19  "DrivMan Steering AngAcc"
  Demux/18 -> BusCreator/18  "DrivMan Steering AngVel"
  Demux/17 -> BusCreator/17  "DrivMan Steering Ang"
  Demux/16 -> BusCreator/16  "DrivMan Gas"
  Demux/15 -> BusCreator/15  "DrivMan Clutch"
  Demux/14 -> BusCreator/14  "DrivMan BrakePark"
  Demux/13 -> BusCreator/13  "DrivMan Brake"
  Demux/12 -> BusCreator/12  "DrivMan GearNo"

== system generic_mass_SoC_mu/CarMaker/IPG Vehicle ==
  Sync_In : Inport
  Vhcl.Model.Source : Inport  Port=2
  VhclCtrl.Steering : Inport  Port=3
  Vhcl.Wheel.In : Inport  Port=4
  Vhcl.Misc : Inport  Port=5
  VhclCtrl.Brake : Inport  Port=6
  VhclCtrl.PT : Inport  Port=7
  Brake : Subsystem
  CarAndTrailer : Subsystem
  PowerTrain : Subsystem
  Stop Simulation : Stop
  VehicleSource_BuiltIn : simulink/Logic and Bit Operations/Compare To Constant  relop=~=  const=1  OutDataTypeStr=boolean  ZeroCross=off
  Sync_Out : Outport  VectorParamsAs1DForOutWhenUnconnected=off
  wires:
  VhclCtrl.PT/1 -> PowerTrain/3(VhclCtrl.PT)
  Brake/1(Sync_Out) -> PowerTrain/1(Sync_In)
  CarAndTrailer/1(Sync_Out) -> Brake/1(Sync_In)
  CarAndTrailer/2(Brake.IF.In) -> Brake/2(Brake.IF.In)
  VhclCtrl.Brake/1 -> Brake/3(VhclCtrl.Brake)
  PowerTrain/1(Sync_Out) -> Sync_Out/1
  Vhcl.Model.Source/1 -> VehicleSource_BuiltIn/1
  VehicleSource_BuiltIn/1 -> Stop Simulation/1
  Brake/2(Vhcl.Wheel.PT) -> PowerTrain/2(Vhcl.Wheel.PT)
  Sync_In/1 -> CarAndTrailer/1(Sync_In)
  VhclCtrl.Steering/1 -> CarAndTrailer/2(VhclCtrl.Steering)
  Vhcl.Wheel.In/1 -> CarAndTrailer/3(Vhcl.Wheel.In)
  Vhcl.Misc/1 -> CarAndTrailer/4(Vhcl.Misc)

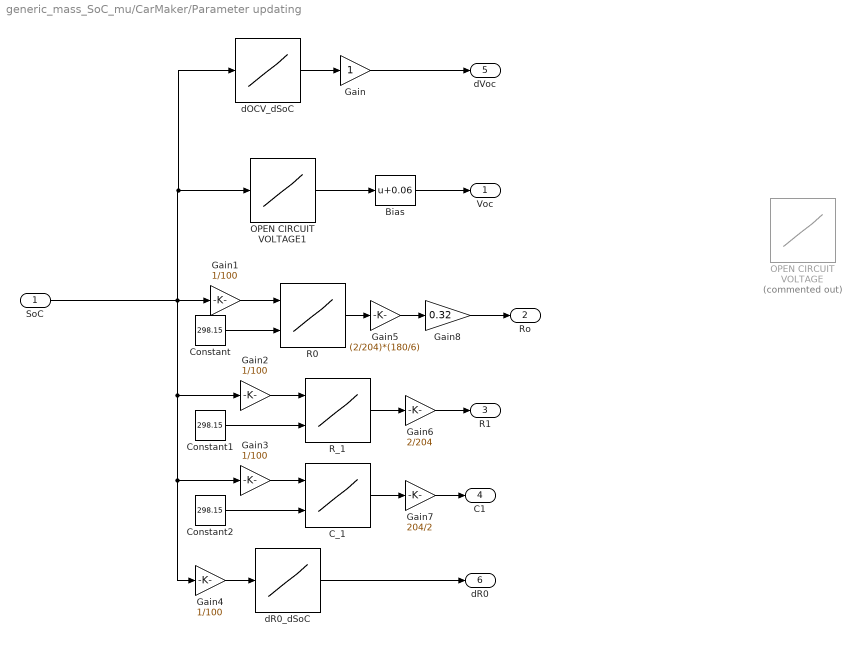
== system generic_mass_SoC_mu/CarMaker/Parameter updating ==
  SoC : Inport
  Bias : Bias  Bias=0.06  SaturateOnIntegerOverflow=off
  C_1 : Lookup_n-D  BreakpointsForDimension1=Battery.SOC_LUT  BreakpointsForDimension2=Battery.Temperature_LUT  Table=Battery.C1_LUT  InternalRulePriority=Speed  RndMeth=Simplest
      settings: InputPortMap=u0,u1
  Constant : Constant  Value=298.15
  Constant1 : Constant  Value=298.15
  Constant2 : Constant  Value=298.15
  Gain : Gain
  Gain{1..4} (4 alike) : Gain  Gain=1/100
  Gain5 : Gain  Gain=(2/204)*(180/6)
  Gain6 : Gain  Gain=2/204
  Gain7 : Gain  Gain=204/2
  Gain8 : Gain  Gain=0.32
  OPEN CIRCUIT VOLTAGE : Lookup_n-D  Commented=on  BreakpointsForDimension1=Battery.SOC_LUT  BreakpointsForDimension2=Battery.Temperature_LUT  Table=Battery.Em_LUT/204  InternalRulePriority=Speed  RndMeth=Simplest
      settings: InputPortMap=u0,u1
  OPEN CIRCUIT VOLTAGE1 : Lookup_n-D  NumberOfTableDimensions=1  BreakpointsForDimension1=Table_SoCvsOCV.LUT.SoC_percent  BreakpointsForDimension2=Battery.Temperature_LUT  Table=Table_SoCvsOCV.LUT.Voltage_V  InternalRulePriority=Speed  RndMeth=Simplest
  R0 : Lookup_n-D  BreakpointsForDimension1=Battery.SOC_LUT  BreakpointsForDimension2=Battery.Temperature_LUT  Table=Battery.R0_LUT  InternalRulePriority=Speed  RndMeth=Simplest
      settings: InputPortMap=u0,u1
  R_1 : Lookup_n-D  BreakpointsForDimension1=Battery.SOC_LUT  BreakpointsForDimension2=Battery.Temperature_LUT  Table=Battery.R1_LUT  InternalRulePriority=Speed  RndMeth=Simplest
      settings: InputPortMap=u0,u1
  dOCV_dSoC : Lookup_n-D  NumberOfTableDimensions=1  BreakpointsForDimension1=SoC_bp  BreakpointsForDimension2=Battery.Temperature_LUT  Table=dOCV_dSoC  InternalRulePriority=Speed  RndMeth=Simplest
  dR0_dSoC : Lookup_n-D  NumberOfTableDimensions=1  BreakpointsForDimension1=SoC_L  BreakpointsForDimension2=Battery.Temperature_LUT  Table=dR0  InternalRulePriority=Speed  RndMeth=Simplest
  Voc : Outport
  Ro : Outport  Port=2
  R1 : Outport  Port=3
  C1 : Outport  Port=4
  dVoc : Outport  Port=5
  dR0 : Outport  Port=6
  wires:
  OPEN CIRCUIT VOLTAGE1/1 -> Bias/1
  dOCV_dSoC/1 -> Gain/1
  Gain/1 -> dVoc/1
  Constant/1 -> R0/2
  Constant1/1 -> R_1/2
  C_1/1 -> Gain7/1
  Constant2/1 -> C_1/2
  SoC/1 -> Gain1/1, Gain2/1, Gain4/1, Gain3/1, OPEN CIRCUIT VOLTAGE1/1, dOCV_dSoC/1
  Gain1/1 -> R0/1
  Gain2/1 -> R_1/1
  Gain3/1 -> C_1/1
  Gain4/1 -> dR0_dSoC/1
  R0/1 -> Gain5/1
  R_1/1 -> Gain6/1
  dR0_dSoC/1 -> dR0/1
  Gain6/1 -> R1/1
  Gain7/1 -> C1/1
  Gain5/1 -> Gain8/1
  Gain8/1 -> Ro/1
  Bias/1 -> Voc/1

== system generic_mass_SoC_mu/CarMaker/RC network subsystem ==
  note: D(V1)
  note: V1
  current (A) : Inport
  R1 : Inport  Port=2
  " C1" : Inport  Port=3
  Discrete-Time Integrator1 : DiscreteIntegrator  SampleTime=-1  ICPrevOutput=DiscIntNeverNeededParam  ICPrevScaledInput=DiscIntNeverNeededParam
  MATLAB Function : MATLAB Function  TreatAsAtomicUnit=on
  V1 : Outport
  wires:
  MATLAB Function/1(y) -> Discrete-Time Integrator1/1
  Discrete-Time Integrator1/1 -> MATLAB Function/4(V1), V1/1
  current (A)/1 -> MATLAB Function/1(I)
  R1/1 -> MATLAB Function/2(R1)
  " C1"/1 -> MATLAB Function/3(C1)

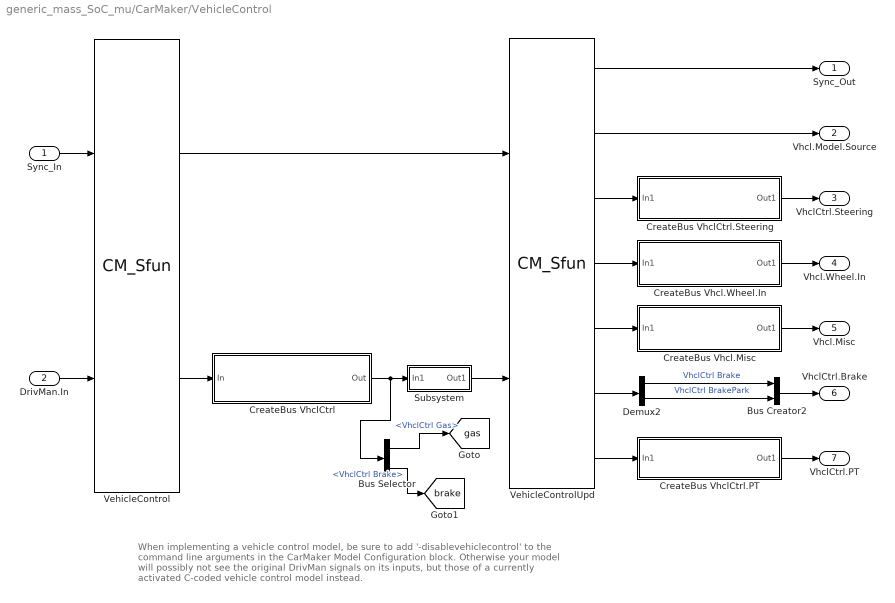
== system generic_mass_SoC_mu/CarMaker/VehicleControl ==
  note: When implementing a vehicle control model,
      | be sure to add '-disablevehiclecontrol' to the command line arguments
      | in the CarMaker Model Configuration block.
      | Otherwise your model will possibly not see the original DrivMan signals
      | on its inputs, but those of a currently activated C-coded vehicle control model instead.
  Sync_In : Inport
  DrivMan.In : Inport  Port=2
  Bus Creator2 : BusCreator  Inputs=2
  Bus Selector : BusSelector  OutputSignals=VhclCtrl Gas,VhclCtrl Brake
  CreateBus Vhcl.Misc : Subsystem
  CreateBus Vhcl.Wheel.In : Subsystem
  CreateBus VhclCtrl : Subsystem
  CreateBus VhclCtrl.PT : Subsystem
  CreateBus VhclCtrl.Steering : Subsystem
  Demux2 : Demux  Outputs=2
      settings: DisplayOption=none
  Subsystem : Subsystem
  VehicleControl : S-Function  FunctionName=CM_Sfun  Parameters='VehicleControl'  SFunctionDeploymentMode=off  EnableBusSupport=off
  VehicleControlUpd : S-Function  FunctionName=CM_Sfun  Parameters='VehicleControlUpd'  SFunctionDeploymentMode=off  EnableBusSupport=off
  Sync_Out : Outport  VectorParamsAs1DForOutWhenUnconnected=off
  Vhcl.Model.Source : Outport  Port=2  VectorParamsAs1DForOutWhenUnconnected=off
  VhclCtrl.Steering : Outport  Port=3  VectorParamsAs1DForOutWhenUnconnected=off
  Vhcl.Wheel.In : Outport  Port=4  VectorParamsAs1DForOutWhenUnconnected=off
  Vhcl.Misc : Outport  Port=5  VectorParamsAs1DForOutWhenUnconnected=off
  VhclCtrl.Brake : Outport  Port=6  VectorParamsAs1DForOutWhenUnconnected=off
  VhclCtrl.PT : Outport  Port=7  VectorParamsAs1DForOutWhenUnconnected=off
  tag scope: brake=global, gas=global
  wires:
  CreateBus VhclCtrl/1(Out) -> Bus Selector/1, Subsystem/1(In1)
  VehicleControl/2 -> CreateBus VhclCtrl/1(In)
  VehicleControlUpd/2 -> Vhcl.Model.Source/1
  VehicleControlUpd/4 -> CreateBus Vhcl.Wheel.In/1(In1)
  VehicleControlUpd/5 -> CreateBus Vhcl.Misc/1(In1)
  VehicleControlUpd/6 -> Demux2/1
  VehicleControlUpd/7 -> CreateBus VhclCtrl.PT/1(In1)
  VehicleControlUpd/3 -> CreateBus VhclCtrl.Steering/1(In1)
  CreateBus Vhcl.Misc/1(Out1) -> Vhcl.Misc/1
  CreateBus Vhcl.Wheel.In/1(Out1) -> Vhcl.Wheel.In/1
  DrivMan.In/1 -> VehicleControl/2
  VehicleControl/1 -> VehicleControlUpd/1
  Sync_In/1 -> VehicleControl/1
  CreateBus VhclCtrl.PT/1(Out1) -> VhclCtrl.PT/1
  Bus Creator2/1 -> VhclCtrl.Brake/1
  CreateBus VhclCtrl.Steering/1(Out1) -> VhclCtrl.Steering/1
  VehicleControlUpd/1 -> Sync_Out/1
  Demux2/2 -> Bus Creator2/2  "VhclCtrl BrakePark"
  Demux2/1 -> Bus Creator2/1  "VhclCtrl Brake"
  Subsystem/1(Out1) -> VehicleControlUpd/2
  Bus Selector/1 -> [gas]  "<VhclCtrl Gas>"
  Bus Selector/2 -> [brake]  "<VhclCtrl Brake>"
